simulink model "DoubleStageRealPred"  (R2019b)
settings: Solver=ode4  StartTime=0.0  StopTime=18  RelTol=1e-3
settings Model: Creator=cwh  LastModifiedBy=cwh

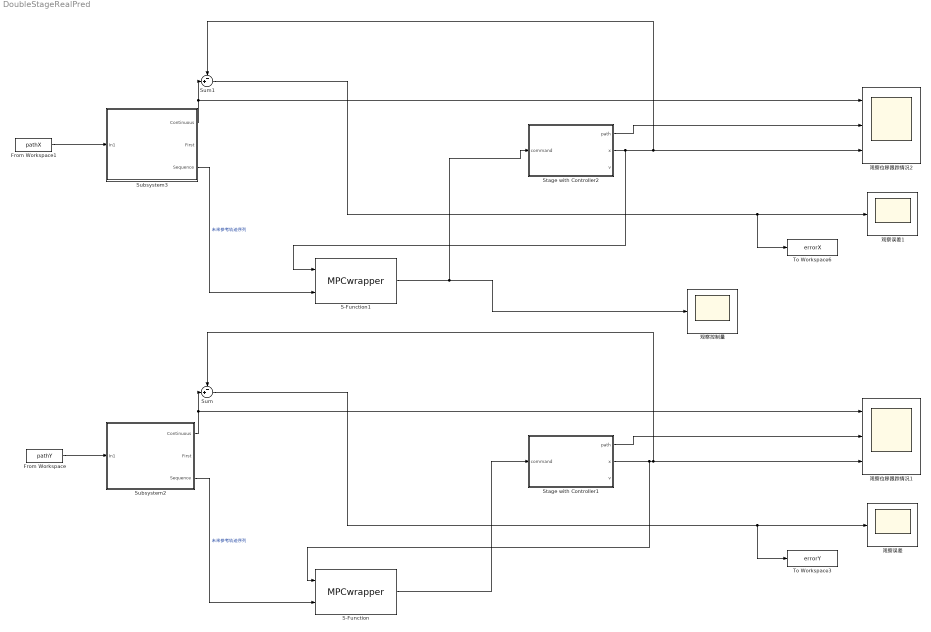
== system DoubleStageRealPred ==
  From Workspace : FromWorkspace  VariableName=pathY
  From Workspace1 : FromWorkspace  VariableName=pathX
  S-Function : S-Function  FunctionName=MPCwrapper  Parameters=ts0,p0,m0,wy0,wu0,pn0,mn0,A0,B0,C0  SFunctionDeploymentMode=off  EnableBusSupport=off  mask{ts0=1/300, p0=10, m0=2, wy0=1, wu0=5, pn0=0.01, mn0=1e-7, A0=[1.0000115706217 0.000609532485011205 -2.90567156941695e-05 -2.8838178802516e-05 -1.32757056614049e-05 6.99601670381165e-06 -3.18120663324485e-06 -2.27814967618556e-05 5.13074986255722e-06 8.75570136392088e-06 4.12216814821496e-05 2.82589511030966e-05 1.38918833632926e-05 -6.77437552299883e-05 2.03141408355556e-05 1.3933401247988e-05;-0.00142090010854529 0.738077101192346 0.122413499211786 -0.137486073360022 0.0313692938010181 -0.0163095393823442 0.0123125504806208 0.0521854309418946 6.06259243465084e-05 -0.0154725457669676 -0.0910984145836639 -0.0623333183109398 -0.0357160274682558 0.166173196031298 -0.0407972392370418 -0.0288592376114164;0.000173836175786984 0.0823796141629645 0.936534129758241 0.129486570923139 -0.036320951241586 0.0361526786601493 -0.0227957163436435 -0.0703897512419776 -0.0143972507608596 0.00891075682097015 0.0708361808080998 0.101081287968089 0.0666029472784014 -0.157648996814292 0.0470342218896352 -0.0399463560456648;-0.000140801564006995 -0.0398995982001749 0.0482178625042528 0.812669889577311 -0.00134999068632695 -0.382616079688584 0.000223178211625097 0.0469231399770238 -0.143810540086395 0.0710128957461141 -0.247834204386692 -0.296513957769691 -0.325210699376732 0.372092331767418 -0.211242033070465 0.293753784515539;3.42470866959143e-05 0.000595695488149375 -9.98528571511104e-05 -0.0458106739318553 -0.533392471426017 0.221623281792913 -0.446616540275579 -0.278237883349058 -0.517847016480996 -0.0278763105014827 -0.294373744139941 0.122216618281759 0.12373803415385 0.219131425654904 0.0115017616869533 -0.201713208121595;-8.38423190414276e-06 -0.000106976325216003 -0.000126356985173674 0.0446104923730838 -0.789330028884095 -0.0635409745139186 0.217315531585003 0.428933672455911 0.380122023748825 0.0118539443720737 0.031851930636314 -0.0414495969904788 -0.023871230040266 0.0546233443229519 0.0196887107193056 0.052104192590526;2.60227374979915e-05 -0.000108118170101408 -0.000165028027829762 -0.108366857314847 0.0486035678395884 -0.812481107087124 -0.383907479476565 0.300783442432763 -0.13042834413557 -0.103189573807195 -0.0565935688344146 -0.0274362100819211 0.0353958321663584 0.134294171065343 0.00317423750621492 -0.111971418132818;-3.04433888484709e-05 -0.000162126560191284 -0.00349103519240706 0.283450286703681 0.0995124872228339 0.158881053680105 -0.727367008574283 0.0203722807986324 0.599675491129193 -0.0144591931777236 -0.117713842477622 -0.214750604757182 -0.143674185220518 0.242363820878842 -0.0424914243896858 0.0399361544437002;-7.03437540239549e-06 0.000673180664052835 -0.000806527449590069 -0.0531789752103619 -0.126210623822268 -0.355796538989817 0.221313903200369 -0.746205189224513 0.390676437840495 -0.0670397603760636 -0.124647984427182 0.143113403041731 0.126491540791009 0.13138458396229 0.0205737838814803 -0.194753468914102;2.94250210549163e-05 0.00380796360407305 -0.00152017446432402 -0.0611450994420722 -0.141604737439109 -0.0621757478962963 -0.0137193325497074 -0.231337973736074 -0.129000060002503 -0.109900722662798 0.346596267960637 -0.6829498818844 0.341397624602706 -0.209809119511644 0.0557623769558337 0.258109813700338;4.16161483004265e-05 -0.00119099502337995 0.00523832742402863 -0.231791036529493 -0.0670769218113561 0.0859917214673652 0.00502321602689937 -0.0819083397585268 0.0258773400195737 -0.921646644786536 0.100187683933086 0.221379072794011 -0.0800944476417409 -0.41793253318707 0.0744399632628906 0.239378893737222;3.8920899086172e-05 0.000182972511262298 0.000644378726536077 -0.037315658616259 -0.103526566385873 -0.00809792406340184 -0.0430927394822072 -0.170484721282916 -0.123227267262762 -0.0230662214508411 0.756729192336082 0.131641548257449 -0.549782659505758 0.210029419700832 0.0128478312282247 -0.159316740319721;-1.23494313607877e-05 0.000741287885504752 -0.0023380433326778 0.159021838335191 0.0203362227220057 -0.0170068380272139 -0.0879225101592911 0.0673806812988783 -0.000157925082430963 -0.0606345146862053 0.372779928663243 0.50648228039986 0.648140884035249 ...(+974 chars)], B0=[0.00435458989019585;-35.2186738169346;6.40433526974319;-0.459394312962695;0.0607951655462246;1.35275426910958;1.50952205753764;-0.00622785385989629;-0.646782757535364;-2.08540665836484;0.245922050634481;-2.61998850314154;-0.149115577921988;1.73297760141929;4.20213931640046;-3.72550416816845], C0=[-6.04701911579492 -0.00171434818466898 3.82341101457957e-05 5.0499819568111e-06 -5.23419383234341e-07 2.20336984254607e-06 -5.90132662307129e-07 -1.86015808653213e-06 -4.31321823868676e-06 -1.13788330355309e-06 -3.67982364484908e-06 -1.4527282762207e-06 4.42330953779436e-06 -4.25178963852947e-07 2.43129704685927e-07 3.3220579642073e-07]}
      mask Display:
      | fprintf('MyMPCinC++');
      | port_label('input', 1, 'mo')
      | port_label('input', 2, 'ref')
      | port_label('output', 1, 'mv')
  S-Function1 : S-Function  FunctionName=MPCwrapper  Parameters=ts0,p0,m0,wy0,wu0,pn0,mn0,A0,B0,C0  SFunctionDeploymentMode=off  EnableBusSupport=off  mask{ts0=1/300, p0=10, m0=2, wy0=1, wu0=5, pn0=0.01, mn0=1e-7, A0=[1.0000115706217 0.000609532485011205 -2.90567156941695e-05 -2.8838178802516e-05 -1.32757056614049e-05 6.99601670381165e-06 -3.18120663324485e-06 -2.27814967618556e-05 5.13074986255722e-06 8.75570136392088e-06 4.12216814821496e-05 2.82589511030966e-05 1.38918833632926e-05 -6.77437552299883e-05 2.03141408355556e-05 1.3933401247988e-05;-0.00142090010854529 0.738077101192346 0.122413499211786 -0.137486073360022 0.0313692938010181 -0.0163095393823442 0.0123125504806208 0.0521854309418946 6.06259243465084e-05 -0.0154725457669676 -0.0910984145836639 -0.0623333183109398 -0.0357160274682558 0.166173196031298 -0.0407972392370418 -0.0288592376114164;0.000173836175786984 0.0823796141629645 0.936534129758241 0.129486570923139 -0.036320951241586 0.0361526786601493 -0.0227957163436435 -0.0703897512419776 -0.0143972507608596 0.00891075682097015 0.0708361808080998 0.101081287968089 0.0666029472784014 -0.157648996814292 0.0470342218896352 -0.0399463560456648;-0.000140801564006995 -0.0398995982001749 0.0482178625042528 0.812669889577311 -0.00134999068632695 -0.382616079688584 0.000223178211625097 0.0469231399770238 -0.143810540086395 0.0710128957461141 -0.247834204386692 -0.296513957769691 -0.325210699376732 0.372092331767418 -0.211242033070465 0.293753784515539;3.42470866959143e-05 0.000595695488149375 -9.98528571511104e-05 -0.0458106739318553 -0.533392471426017 0.221623281792913 -0.446616540275579 -0.278237883349058 -0.517847016480996 -0.0278763105014827 -0.294373744139941 0.122216618281759 0.12373803415385 0.219131425654904 0.0115017616869533 -0.201713208121595;-8.38423190414276e-06 -0.000106976325216003 -0.000126356985173674 0.0446104923730838 -0.789330028884095 -0.0635409745139186 0.217315531585003 0.428933672455911 0.380122023748825 0.0118539443720737 0.031851930636314 -0.0414495969904788 -0.023871230040266 0.0546233443229519 0.0196887107193056 0.052104192590526;2.60227374979915e-05 -0.000108118170101408 -0.000165028027829762 -0.108366857314847 0.0486035678395884 -0.812481107087124 -0.383907479476565 0.300783442432763 -0.13042834413557 -0.103189573807195 -0.0565935688344146 -0.0274362100819211 0.0353958321663584 0.134294171065343 0.00317423750621492 -0.111971418132818;-3.04433888484709e-05 -0.000162126560191284 -0.00349103519240706 0.283450286703681 0.0995124872228339 0.158881053680105 -0.727367008574283 0.0203722807986324 0.599675491129193 -0.0144591931777236 -0.117713842477622 -0.214750604757182 -0.143674185220518 0.242363820878842 -0.0424914243896858 0.0399361544437002;-7.03437540239549e-06 0.000673180664052835 -0.000806527449590069 -0.0531789752103619 -0.126210623822268 -0.355796538989817 0.221313903200369 -0.746205189224513 0.390676437840495 -0.0670397603760636 -0.124647984427182 0.143113403041731 0.126491540791009 0.13138458396229 0.0205737838814803 -0.194753468914102;2.94250210549163e-05 0.00380796360407305 -0.00152017446432402 -0.0611450994420722 -0.141604737439109 -0.0621757478962963 -0.0137193325497074 -0.231337973736074 -0.129000060002503 -0.109900722662798 0.346596267960637 -0.6829498818844 0.341397624602706 -0.209809119511644 0.0557623769558337 0.258109813700338;4.16161483004265e-05 -0.00119099502337995 0.00523832742402863 -0.231791036529493 -0.0670769218113561 0.0859917214673652 0.00502321602689937 -0.0819083397585268 0.0258773400195737 -0.921646644786536 0.100187683933086 0.221379072794011 -0.0800944476417409 -0.41793253318707 0.0744399632628906 0.239378893737222;3.8920899086172e-05 0.000182972511262298 0.000644378726536077 -0.037315658616259 -0.103526566385873 -0.00809792406340184 -0.0430927394822072 -0.170484721282916 -0.123227267262762 -0.0230662214508411 0.756729192336082 0.131641548257449 -0.549782659505758 0.210029419700832 0.0128478312282247 -0.159316740319721;-1.23494313607877e-05 0.000741287885504752 -0.0023380433326778 0.159021838335191 0.0203362227220057 -0.0170068380272139 -0.0879225101592911 0.0673806812988783 -0.000157925082430963 -0.0606345146862053 0.372779928663243 0.50648228039986 0.648140884035249 ...(+974 chars)], B0=[0.00435458989019585;-35.2186738169346;6.40433526974319;-0.459394312962695;0.0607951655462246;1.35275426910958;1.50952205753764;-0.00622785385989629;-0.646782757535364;-2.08540665836484;0.245922050634481;-2.61998850314154;-0.149115577921988;1.73297760141929;4.20213931640046;-3.72550416816845], C0=[-6.04701911579492 -0.00171434818466898 3.82341101457957e-05 5.0499819568111e-06 -5.23419383234341e-07 2.20336984254607e-06 -5.90132662307129e-07 -1.86015808653213e-06 -4.31321823868676e-06 -1.13788330355309e-06 -3.67982364484908e-06 -1.4527282762207e-06 4.42330953779436e-06 -4.25178963852947e-07 2.43129704685927e-07 3.3220579642073e-07]}
      mask Display:
      | fprintf('MyMPCinC++');
      | port_label('input', 1, 'mo')
      | port_label('input', 2, 'ref')
      | port_label('output', 1, 'mv')
  Stage with Controller1 : Subsystem  mask{tc=1/300, ts=5e-5, vm=0.5, am=3}
      mask prompts: tc "Command period"; ts "Servoing period"; vm "vmax"; am "amax"
  Stage with Controller2 : Subsystem  mask{tc=1/300, ts=5e-5, vm=0.5, am=3}
      mask prompts: tc "Command period"; ts "Servoing period"; vm "vmax"; am "amax"
  Subsystem2 : Subsystem  mask{tc=1/300, p=10}
      mask prompts: tc "Control period"; p "Preview Length"
  Subsystem3 : Subsystem  mask{tc=1/300, p=10}
      mask prompts: tc "Control period"; p "Preview Length"
  Sum : Sum  Inputs=-+|
  Sum1 : Sum  Inputs=-+|
  To Workspace3 : ToWorkspace  VariableName=errorY  SampleTime=1/300
      settings: Save2DSignal=2-D array (concatenate along first dimension)
  To Workspace6 : ToWorkspace  VariableName=errorX  SampleTime=1/300
      settings: Save2DSignal=2-D array (concatenate along first dimension)
  观察位移跟踪情况1 : Scope  NumInputPorts=3
  观察位移跟踪情况2 : Scope  NumInputPorts=3
  观察控制量 : Scope
  观察误差 : Scope
  观察误差1 : Scope
  wires:
  From Workspace/1 -> Subsystem2/1(In1)
  Subsystem2/3(Sequence) -> S-Function/2  "未来参考轨迹序列"
  Stage with Controller1/2(x) -> S-Function/1, Sum/1, 观察位移跟踪情况1/3
  Sum/1 -> To Workspace3/1, 观察误差/1
  Stage with Controller1/1(path) -> 观察位移跟踪情况1/2
  Subsystem2/1(Continuous) -> 观察位移跟踪情况1/1, Sum/2
  Stage with Controller2/2(x) -> 观察位移跟踪情况2/3, Sum1/1, S-Function1/1
  Subsystem3/1(Continuous) -> 观察位移跟踪情况2/1, Sum1/2
  Stage with Controller2/1(path) -> 观察位移跟踪情况2/2
  Sum1/1 -> To Workspace6/1, 观察误差1/1
  From Workspace1/1 -> Subsystem3/1(In1)
  Subsystem3/3(Sequence) -> S-Function1/2  "未来参考轨迹序列"
  S-Function1/1 -> 观察控制量/1, Stage with Controller2/1(command)
  S-Function/1 -> Stage with Controller1/1(command)

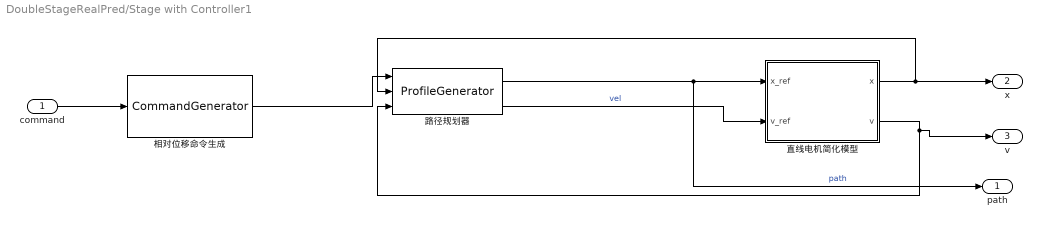
== system DoubleStageRealPred/Stage with Controller1 ==
  command : Inport
  直线电机简化模型 : Subsystem  mask{ts=ts, L=1.94e-3, R=2.46, Ki=4.6, Kf=0, Kbemf=2.81, M=1, Kpx=15, Kix=0.001, Kdx=0.02, Kpv=0.05, Kiv=0.5, Kdv=0, Kpi=5, Kii=0.0015, Kdi=0}
      mask prompts: ts "Servoing period"; L "Coil inductance"; R "Coil resistance"; Ki "Force coefficient"; Kf "Friction coefficient"; Kbemf "Back EMF Coefficient"; M "Moving mass"; Kpx "Kp in position loop"; Kix "Ki in position loop"; Kdx "Kd in position loop"; Kpv "Kp in velocity loop"; Kiv "Ki in velocity lpop"; Kdv "Kd in velocity loop"; Kpi "Kp in current loop"; Kii "Ki in current loop"; Kdi "Kd in current loop"
  相对位移命令生成 : S-Function  FunctionName=CommandGenerator  Parameters=ts0,cp0  SFunctionDeploymentMode=off  EnableBusSupport=off  mask{ts0=ts, cp0=tc}
      mask prompts: ts0 "Serving period"; cp0 "Command period"
  路径规划器 : S-Function  FunctionName=ProfileGenerator  Parameters=ts0,vmax0,amax0  SFunctionDeploymentMode=off  EnableBusSupport=off  mask{ts0=ts, vmax0=vm, amax0=am}
      mask prompts: ts0 "Servoing period"; vmax0 "Max velocity"; amax0 "Max acceleration"
  path : Outport
  x : Outport  Port=2
  v : Outport  Port=3
  wires:
  路径规划器/2 -> 直线电机简化模型/2(v_ref)  "vel"
  路径规划器/1 -> path/1, 直线电机简化模型/1(x_ref)  "path"
  直线电机简化模型/1(x) -> 路径规划器/2, x/1
  command/1 -> 相对位移命令生成/1
  相对位移命令生成/1 -> 路径规划器/1
  直线电机简化模型/2(v) -> 路径规划器/3, v/1

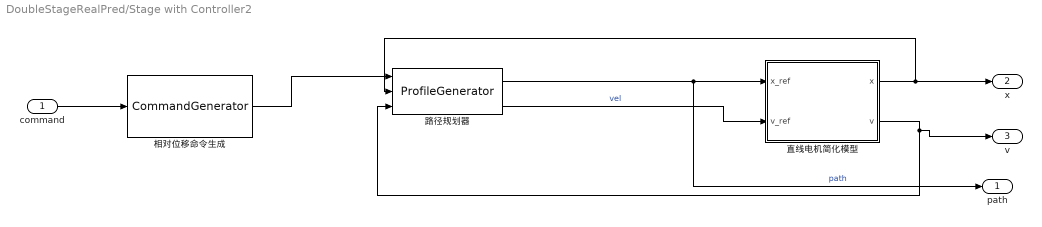
== system DoubleStageRealPred/Stage with Controller2 ==
  command : Inport
  直线电机简化模型 : Subsystem  mask{ts=ts, L=1.94e-3, R=2.46, Ki=4.6, Kf=0, Kbemf=2.81, M=1, Kpx=15, Kix=0.001, Kdx=0.02, Kpv=0.05, Kiv=0.5, Kdv=0, Kpi=5, Kii=0.0015, Kdi=0}
      mask prompts: ts "Servoing period"; L "Coil inductance"; R "Coil resistance"; Ki "Force coefficient"; Kf "Friction coefficient"; Kbemf "Back EMF Coefficient"; M "Moving mass"; Kpx "Kp in position loop"; Kix "Ki in position loop"; Kdx "Kd in position loop"; Kpv "Kp in velocity loop"; Kiv "Ki in velocity lpop"; Kdv "Kd in velocity loop"; Kpi "Kp in current loop"; Kii "Ki in current loop"; Kdi "Kd in current loop"
  相对位移命令生成 : S-Function  FunctionName=CommandGenerator  Parameters=ts0,cp0  SFunctionDeploymentMode=off  EnableBusSupport=off  mask{ts0=ts, cp0=tc}
      mask prompts: ts0 "Serving period"; cp0 "Command period"
  路径规划器 : S-Function  FunctionName=ProfileGenerator  Parameters=ts0,vmax0,amax0  SFunctionDeploymentMode=off  EnableBusSupport=off  mask{ts0=ts, vmax0=vm, amax0=am}
      mask prompts: ts0 "Servoing period"; vmax0 "Max velocity"; amax0 "Max acceleration"
  path : Outport
  x : Outport  Port=2
  v : Outport  Port=3
  wires:
  路径规划器/2 -> 直线电机简化模型/2(v_ref)  "vel"
  路径规划器/1 -> path/1, 直线电机简化模型/1(x_ref)  "path"
  直线电机简化模型/1(x) -> 路径规划器/2, x/1
  command/1 -> 相对位移命令生成/1
  相对位移命令生成/1 -> 路径规划器/1
  直线电机简化模型/2(v) -> 路径规划器/3, v/1

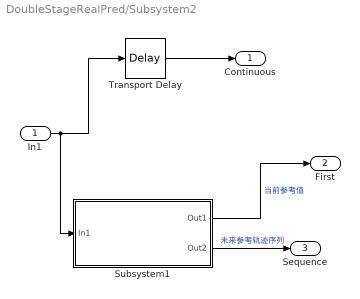
== system DoubleStageRealPred/Subsystem2 ==
  In1 : Inport
  Subsystem1 : Subsystem  mask{ts0=tc, length0=p}
      mask prompts: ts0 "Sample time"; length0 "Preview length"
      mask Display:
      | fprintf('Reference\nPreviewer');
      | port_label('input', 1, 'input')
      | port_label('output', 1, 'first')
      | port_label('output', 2, 'seq')
  Transport Delay : TransportDelay  DelayTime=tc*p  BufferSize=2048
  Continuous : Outport
  First : Outport  Port=2
  Sequence : Outport  Port=3
  wires:
  In1/1 -> Subsystem1/1(In1), Transport Delay/1
  Transport Delay/1 -> Continuous/1
  Subsystem1/1(Out1) -> First/1  "当前参考值"
  Subsystem1/2(Out2) -> Sequence/1  "未来参考轨迹序列"

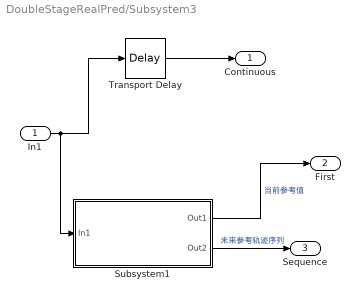
== system DoubleStageRealPred/Subsystem3 ==
  In1 : Inport
  Subsystem1 : Subsystem  mask{ts0=tc, length0=p}
      mask prompts: ts0 "Sample time"; length0 "Preview length"
      mask Display:
      | fprintf('Reference\nPreviewer');
      | port_label('input', 1, 'input')
      | port_label('output', 1, 'first')
      | port_label('output', 2, 'seq')
  Transport Delay : TransportDelay  DelayTime=tc*p  BufferSize=2048
  Continuous : Outport
  First : Outport  Port=2
  Sequence : Outport  Port=3
  wires:
  In1/1 -> Subsystem1/1(In1), Transport Delay/1
  Transport Delay/1 -> Continuous/1
  Subsystem1/1(Out1) -> First/1  "当前参考值"
  Subsystem1/2(Out2) -> Sequence/1  "未来参考轨迹序列"

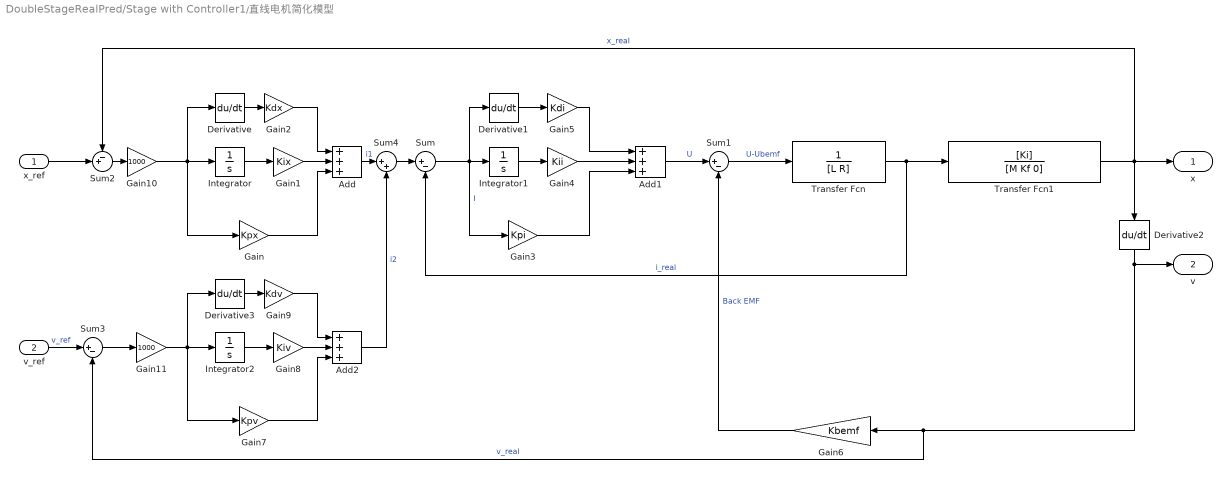
== system DoubleStageRealPred/Stage with Controller1/直线电机简化模型 ==
  x_ref : Inport
  v_ref : Inport  Port=2
  Add : Sum  Inputs=+++
  Add1 : Sum  Inputs=+++
  Add2 : Sum  Inputs=+++
  Derivative{,1..3} (4 alike) : Derivative
  Gain : Gain  Gain=Kpx
  Gain1 : Gain  Gain=Kix
  Gain10 : Gain  Gain=1000
  Gain11 : Gain  Gain=1000
  Gain2 : Gain  Gain=Kdx
  Gain3 : Gain  Gain=Kpi
  Gain4 : Gain  Gain=Kii
  Gain5 : Gain  Gain=Kdi
  Gain6 : Gain  Gain=Kbemf
  Gain7 : Gain  Gain=Kpv
  Gain8 : Gain  Gain=Kiv
  Gain9 : Gain  Gain=Kdv
  Integrator : Integrator
  Integrator1 : Integrator
  Integrator2 : Integrator
  Sum : Sum  Inputs=|+-
  Sum1 : Sum  Inputs=|+-
  Sum2 : Sum  Inputs=-+|
  Sum3 : Sum  Inputs=|+-
  Sum4 : Sum  Inputs=|++
  Transfer Fcn : TransferFcn  Denominator=[L R]
  Transfer Fcn1 : TransferFcn  Numerator=[Ki]  Denominator=[M Kf 0]
  x : Outport
  v : Outport  Port=2
  wires:
  Gain10/1 -> Derivative/1, Gain/1, Integrator/1
  Derivative/1 -> Gain2/1
  Integrator/1 -> Gain1/1
  Gain2/1 -> Add/1
  Gain1/1 -> Add/2
  Gain/1 -> Add/3
  Sum/1 -> Derivative1/1, Gain3/1, Integrator1/1  "I"
  Gain3/1 -> Add1/3
  Gain4/1 -> Add1/2
  Integrator1/1 -> Gain4/1
  Gain5/1 -> Add1/1
  Derivative1/1 -> Gain5/1
  Add1/1 -> Sum1/1  "U"
  Transfer Fcn/1 -> Transfer Fcn1/1, Sum/2  "i_real"
  Sum1/1 -> Transfer Fcn/1  "U-Ubemf"
  Transfer Fcn1/1 -> x/1, Sum2/1, Derivative2/1  "x_reaI"
  Derivative2/1 -> v/1, Sum3/2, Gain6/1  "v_real"
  Gain6/1 -> Sum1/2  "Back EMF"
  Gain7/1 -> Add2/3
  Gain11/1 -> Derivative3/1, Gain7/1, Integrator2/1
  Gain8/1 -> Add2/2
  Integrator2/1 -> Gain8/1
  Add2/1 -> Sum4/2  "i2"
  Gain9/1 -> Add2/1
  Derivative3/1 -> Gain9/1
  v_ref/1 -> Sum3/1  "v_ref"
  Add/1 -> Sum4/1  "i1"
  Sum4/1 -> Sum/1
  x_ref/1 -> Sum2/2
  Sum3/1 -> Gain11/1
  Sum2/1 -> Gain10/1

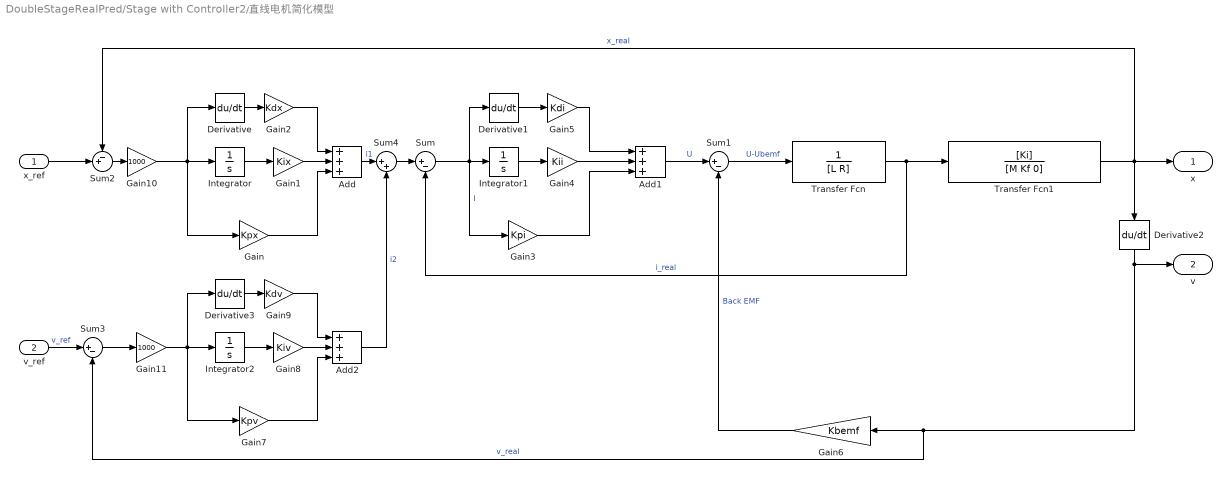
== system DoubleStageRealPred/Stage with Controller2/直线电机简化模型 ==
  x_ref : Inport
  v_ref : Inport  Port=2
  Add : Sum  Inputs=+++
  Add1 : Sum  Inputs=+++
  Add2 : Sum  Inputs=+++
  Derivative{,1..3} (4 alike) : Derivative
  Gain : Gain  Gain=Kpx
  Gain1 : Gain  Gain=Kix
  Gain10 : Gain  Gain=1000
  Gain11 : Gain  Gain=1000
  Gain2 : Gain  Gain=Kdx
  Gain3 : Gain  Gain=Kpi
  Gain4 : Gain  Gain=Kii
  Gain5 : Gain  Gain=Kdi
  Gain6 : Gain  Gain=Kbemf
  Gain7 : Gain  Gain=Kpv
  Gain8 : Gain  Gain=Kiv
  Gain9 : Gain  Gain=Kdv
  Integrator : Integrator
  Integrator1 : Integrator
  Integrator2 : Integrator
  Sum : Sum  Inputs=|+-
  Sum1 : Sum  Inputs=|+-
  Sum2 : Sum  Inputs=-+|
  Sum3 : Sum  Inputs=|+-
  Sum4 : Sum  Inputs=|++
  Transfer Fcn : TransferFcn  Denominator=[L R]
  Transfer Fcn1 : TransferFcn  Numerator=[Ki]  Denominator=[M Kf 0]
  x : Outport
  v : Outport  Port=2
  wires:
  Gain10/1 -> Derivative/1, Gain/1, Integrator/1
  Derivative/1 -> Gain2/1
  Integrator/1 -> Gain1/1
  Gain2/1 -> Add/1
  Gain1/1 -> Add/2
  Gain/1 -> Add/3
  Sum/1 -> Derivative1/1, Gain3/1, Integrator1/1  "I"
  Gain3/1 -> Add1/3
  Gain4/1 -> Add1/2
  Integrator1/1 -> Gain4/1
  Gain5/1 -> Add1/1
  Derivative1/1 -> Gain5/1
  Add1/1 -> Sum1/1  "U"
  Transfer Fcn/1 -> Transfer Fcn1/1, Sum/2  "i_real"
  Sum1/1 -> Transfer Fcn/1  "U-Ubemf"
  Transfer Fcn1/1 -> x/1, Sum2/1, Derivative2/1  "x_reaI"
  Derivative2/1 -> v/1, Sum3/2, Gain6/1  "v_real"
  Gain6/1 -> Sum1/2  "Back EMF"
  Gain7/1 -> Add2/3
  Gain11/1 -> Derivative3/1, Gain7/1, Integrator2/1
  Gain8/1 -> Add2/2
  Integrator2/1 -> Gain8/1
  Add2/1 -> Sum4/2  "i2"
  Gain9/1 -> Add2/1
  Derivative3/1 -> Gain9/1
  v_ref/1 -> Sum3/1  "v_ref"
  Add/1 -> Sum4/1  "i1"
  Sum4/1 -> Sum/1
  x_ref/1 -> Sum2/2
  Sum3/1 -> Gain11/1
  Sum2/1 -> Gain10/1

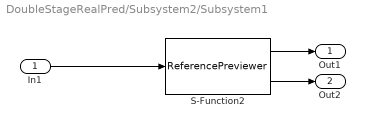
== system DoubleStageRealPred/Subsystem2/Subsystem1 ==
  In1 : Inport
  S-Function2 : S-Function  FunctionName=ReferencePreviewer  Parameters=tc,p  SFunctionDeploymentMode=off  EnableBusSupport=off
  Out1 : Outport  VectorParamsAs1DForOutWhenUnconnected=off
  Out2 : Outport  Port=2  VectorParamsAs1DForOutWhenUnconnected=off
  wires:
  S-Function2/1 -> Out1/1
  S-Function2/2 -> Out2/1
  In1/1 -> S-Function2/1

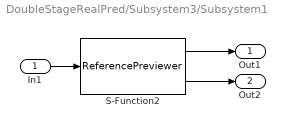
== system DoubleStageRealPred/Subsystem3/Subsystem1 ==
  In1 : Inport
  S-Function2 : S-Function  FunctionName=ReferencePreviewer  Parameters=tc,p  SFunctionDeploymentMode=off  EnableBusSupport=off
  Out1 : Outport  VectorParamsAs1DForOutWhenUnconnected=off
  Out2 : Outport  Port=2  VectorParamsAs1DForOutWhenUnconnected=off
  wires:
  S-Function2/1 -> Out1/1
  S-Function2/2 -> Out2/1
  In1/1 -> S-Function2/1
